simulink model "NE_Red_Rooster_Delta_B_28may"  (R2019b)
settings: Solver=FixedStepAuto  StartTime=0.0  StopTime=inf  FixedStep=0.0005  RelTol=1e-3
PreLoadFcn:
  | waijung.modelPreload; % Required for working with Waijung Blockset. Do not remove.
undefined symbols (not defined in the file): ARM, DiscIntNeverNeededParam, HSEOSC, Link, LQFP100, MDK, ST, STM32F407VG
libraries: simulink x30, stm32f4_i2c_lib x22, stm32f4_io_lib x6, stm32f4_reset_lib x1, stm32f4_device_config_lib x1
(part 3 of 5)

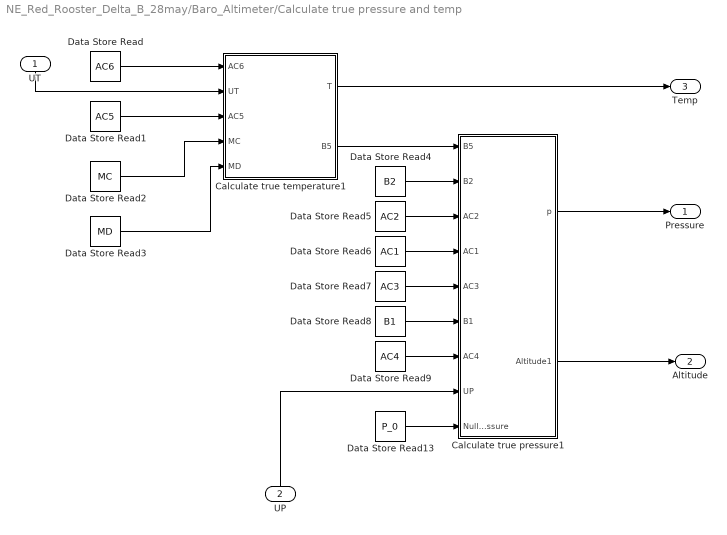
== system NE_Red_Rooster_Delta_B_28may/Baro_Altimeter/Calculate true pressure and temp  ==
  UT : Inport
  "UP " : Inport  Port=2
  Calculate true pressure1 : Subsystem
  Calculate true temperature1 : Subsystem
  Data Store Read : DataStoreRead  DataStoreName=AC6
  Data Store Read1 : DataStoreRead  DataStoreName=AC5
  Data Store Read13 : DataStoreRead  DataStoreName=P_0
  Data Store Read2 : DataStoreRead  DataStoreName=MC
  Data Store Read3 : DataStoreRead  DataStoreName=MD
  Data Store Read4 : DataStoreRead  DataStoreName=B2
  Data Store Read5 : DataStoreRead  DataStoreName=AC2
  Data Store Read6 : DataStoreRead  DataStoreName=AC1
  Data Store Read7 : DataStoreRead  DataStoreName=AC3
  Data Store Read8 : DataStoreRead  DataStoreName=B1
  Data Store Read9 : DataStoreRead  DataStoreName=AC4
  Pressure : Outport
  Altitude : Outport  Port=2
  "Temp " : Outport  Port=3
  wires:
  Calculate true temperature1/2(B5) -> Calculate true pressure1/1(B5)
  Calculate true pressure1/1(p) -> Pressure/1
  Calculate true pressure1/2(Altitude1) -> Altitude/1
  Data Store Read/1 -> Calculate true temperature1/1(AC6)
  Data Store Read1/1 -> Calculate true temperature1/3(AC5)
  Data Store Read2/1 -> Calculate true temperature1/4(MC)
  Data Store Read3/1 -> Calculate true temperature1/5(MD)
  Data Store Read4/1 -> Calculate true pressure1/2(B2)
  Data Store Read5/1 -> Calculate true pressure1/3(AC2)
  Data Store Read6/1 -> Calculate true pressure1/4(AC1)
  Data Store Read7/1 -> Calculate true pressure1/5(AC3)
  Data Store Read8/1 -> Calculate true pressure1/6(B1)
  Data Store Read9/1 -> Calculate true pressure1/7(AC4)
  Calculate true temperature1/1(T) -> "Temp "/1
  Data Store Read13/1 -> Calculate true pressure1/9("Null_Pressure ")
  "UP "/1 -> Calculate true pressure1/8(UP)
  UT/1 -> Calculate true temperature1/2(UT)

== system NE_Red_Rooster_Delta_B_28may/Baro_Altimeter/Read Pressure and Temp ==
  Constant : Constant  Value=hex2dec('EE')  OutDataTypeStr=uint8  SampleTime=-1
  Constant1 : Constant  Value=hex2dec('F4')  OutDataTypeStr=uint8  SampleTime=-1
  Constant4 : Constant  Value=hex2dec('2E')  OutDataTypeStr=uint8  SampleTime=-1
  Constant7 : Constant  Value=hex2dec('B4')  OutDataTypeStr=uint8  SampleTime=-1
  I2C Master Read/Write : stm32f4_i2c_lib/I2C Master Read//Write  configuration=Transaction  module=1  lastmodule=3  transfer=Blocking  dutycycle=TLow/THigh = 2  clkspeed=400  timeout=25  writecount=2  readcount=0  sdapin=C9  sclpin=A8  waitwritetime=14  forcestop=off  inputtypearray=[3 3 3 3]  outputtypearray=[1 3]  confstr="[\"C\",\"9\",\"A\",\"8\",\"1\",\"1\",\"6\",\"0\",\"I2C_DutyCycle_2\",\"14\",\"off\"]"  sampletime=-1  sampletimestr=-1  blockid=Baro_AltimeterReadPressureandTempI2CMasterReadWrite
  I2C Master Read/Write1 : stm32f4_i2c_lib/I2C Master Read//Write  configuration=Transaction  module=1  lastmodule=3  transfer=Blocking  dutycycle=TLow/THigh = 2  clkspeed=400  timeout=25  writecount=2  readcount=0  sdapin=C9  sclpin=A8  waitwritetime=5  forcestop=off  inputtypearray=[3 3 3 3]  outputtypearray=[1 3]  confstr="[\"C\",\"9\",\"A\",\"8\",\"1\",\"1\",\"6\",\"0\",\"I2C_DutyCycle_2\",\"5\",\"off\"]"  sampletime=-1  sampletimestr=-1  blockid=Baro_AltimeterReadPressureandTempI2CMasterReadWrite1
  If : If  IfExpression=u1 == 0  ShowElse=off
  If Action Subsystem : Subsystem  TreatAsAtomicUnit=on
  If Action Subsystem2 : Subsystem  TreatAsAtomicUnit=on
  If2 : If  IfExpression=u1 == 0  ShowElse=off
  UT : Outport
  UP : Outport  Port=2  OutDataTypeStr=uint32
  wires:
  Constant4/1 -> I2C Master Read/Write1/3
  If/1 -> If Action Subsystem/Action
  I2C Master Read/Write1/1 -> If/1
  If2/1 -> If Action Subsystem2/Action
  I2C Master Read/Write/1 -> If2/1
  Constant/1 -> I2C Master Read/Write/1, I2C Master Read/Write1/1
  Constant1/1 -> I2C Master Read/Write/2, I2C Master Read/Write1/2
  Constant7/1 -> I2C Master Read/Write/3
  If Action Subsystem2/1(Out1) -> UP/1
  If Action Subsystem/1(Out1) -> UT/1

== system NE_Red_Rooster_Delta_B_28may/Baro_Altimeter/Subsystem1 ==
  In1 : Inport
  Enable : EnablePort
  Constant : Constant  Value=0
  Data Store Write : DataStoreWrite  DataStoreName=P_0
  Data Store Write1 : DataStoreWrite
  wires:
  Constant/1 -> Data Store Write1/1
  In1/1 -> Data Store Write/1

== system NE_Red_Rooster_Delta_B_28may/Calibration data/Read calibration data  ==
  Subsystem_get_AC : Subsystem
  Subsystem_get_B : Subsystem
  Subsystem_get_M : Subsystem
  AC1 : Outport  OutDataTypeStr=int32
  AC2 : Outport  Port=2  OutDataTypeStr=int32
  AC3 : Outport  Port=3  OutDataTypeStr=int32
  AC4 : Outport  Port=4  OutDataTypeStr=uint32
  AC5 : Outport  Port=5  OutDataTypeStr=uint32
  AC6 : Outport  Port=6
  B1 : Outport  Port=7  OutDataTypeStr=int32
  B2 : Outport  Port=8  OutDataTypeStr=int32
  MB : Outport  Port=9  OutDataTypeStr=int32
  MC : Outport  Port=10  OutDataTypeStr=int32
  MD : Outport  Port=11  OutDataTypeStr=int32
  wires:
  Subsystem_get_M/1(MB) -> MB/1
  Subsystem_get_M/2(MC) -> MC/1
  Subsystem_get_M/3(MD) -> MD/1
  Subsystem_get_B/1(B1) -> B1/1
  Subsystem_get_B/2(B2) -> B2/1
  Subsystem_get_AC/6(AC6) -> AC6/1
  Subsystem_get_AC/5(AC5) -> AC5/1
  Subsystem_get_AC/4(AC4) -> AC4/1
  Subsystem_get_AC/3(AC3) -> AC3/1
  Subsystem_get_AC/2(AC2) -> AC2/1
  Subsystem_get_AC/1(AC1) -> AC1/1

== system NE_Red_Rooster_Delta_B_28may/Elevons_Throttle_PWM/If Action Subsystem ==
  In1 : Inport
  In2 : Inport  Port=2
  In3 : Inport  Port=3
  Action Port : ActionPort  ActionPortLabel=if { }
  Out1 : Outport
  Out2 : Outport  Port=2
  Out3 : Outport  Port=3
  wires:
  In1/1 -> Out1/1
  In2/1 -> Out2/1
  In3/1 -> Out3/1

== system NE_Red_Rooster_Delta_B_28may/Elevons_Throttle_PWM/If Action Subsystem2 ==
  In1 : Inport
  In2 : Inport  Port=2
  In3 : Inport  Port=3
  Action Port : ActionPort  ActionPortLabel=if { }
  Out1 : Outport
  Out2 : Outport  Port=2
  Out3 : Outport  Port=3
  wires:
  In1/1 -> Out1/1
  In2/1 -> Out2/1
  In3/1 -> Out3/1

== system NE_Red_Rooster_Delta_B_28may/Elevons_Throttle_PWM/If Action Subsystem3 ==
  In1 : Inport
  In2 : Inport  Port=2
  In3 : Inport  Port=3
  Action Port : ActionPort  ActionPortLabel=if { }
  Out1 : Outport
  Out2 : Outport  Port=2
  Out3 : Outport  Port=3
  wires:
  In3/1 -> Out3/1
  In2/1 -> Out2/1
  In1/1 -> Out1/1

== system NE_Red_Rooster_Delta_B_28may/Init_ADXL345/Subsystem ==
  Enable : EnablePort
  Constant : Constant
  Out1 : Outport
  wires:
  Constant/1 -> Out1/1

== system NE_Red_Rooster_Delta_B_28may/Init_L3GD4200 /Get Init L3G4200D1 ==
  SlvAddr : Inport
  Bitwise Operator : simulink/Logic and Bit Operations/Bitwise Operator  logicop=AND  UseBitMask=off  NumInputPorts=4  BitMask=bin2dec('11011001')  BitMaskRealWorld=Stored Integer
  CNTRL_REG1 : Constant  Value=hex2dec('20')  OutDataTypeStr=uint8  SampleTime=-1
  CNTRL_REG4 : Constant  Value=hex2dec('23')  OutDataTypeStr=uint8  SampleTime=-1
  Compare To Constant : simulink/Logic and Bit Operations/Compare To Constant  relop===  const=0  OutDataTypeStr=uint8  ZeroCross=off
  Compare To Constant1 : simulink/Logic and Bit Operations/Compare To Constant  relop===  const=hex2dec('0F')  OutDataTypeStr=uint8  ZeroCross=off
  Compare To Constant2 : simulink/Logic and Bit Operations/Compare To Constant  relop===  const=0  OutDataTypeStr=uint8  ZeroCross=off
  Compare To Constant3 : simulink/Logic and Bit Operations/Compare To Constant  relop===  const=0  OutDataTypeStr=uint8  ZeroCross=off
  I2C Master Read/Write : S-Function  FunctionName=stm32f4_i2c  Parameters=configuration,module,transfer,clkspeed,timeout,sdapin,sclpin,writecount,readcount,inputtypearray,outputtypearray,confstr,sampletime,sampletimestr,blockid  SFunctionDeploymentMode=off  EnableBusSupport=off  mask(stm32f4_i2c){configuration=Transaction, module=1, lastmodule=3, transfer=Blocking, dutycycle=TLow/THigh = 2, clkspeed=400, timeout=25, writecount=1, readcount=1, sdapin=C9, sclpin=A8, waitwritetime=0, inputtypearray=[2 3 3], outputtypearray=[2 3 3], confstr=["C","9","A","8","1","1","6","0","I2C_DutyCycle_2","0","off"], sampletime=-1, sampletimestr=0.0005, blockid=Init_L3GD4200GetInitL3G4200D1I2CMasterReadWrite}
      mask prompts: module "I2C Module"; lastmodule "Last module"; transfer "Transfer mode"; dutycycle "Duty cycle in fast mode"; clkspeed "Clock speed (kHz)"; timeout "Timeout (ms)"; writecount "Bytes write count"; readcount "Bytes read count"; sdapin "SDA pin"; sclpin "SCL pin"; waitwritetime "Wait write time (ms), default is 0"; inputtypearray "Input type array"; outputtypearray "Output type array"; confstr "Configuration string"; sampletime "Sample time (sec)"; sampletimestr "Compiled sample time (sec) in string"
      mask init:
      | stm32f4_i2c_callback('init');
      mask Help: web(fullfile(waijungdocroot,'stm32f4_i2c.htm'), '-browser')
      mask TypeOptions configuration: Setup | Transaction
      mask Callback configuration: stm32f4_i2c_callback('configuration');
      mask TypeOptions module: 1 | 2 | 3
      mask Callback module: stm32f4_i2c_callback('module');
      mask TypeOptions transfer: Blocking | Non-blocking
      mask TypeOptions dutycycle: TLow/THigh = 16/9 | TLow/THigh = 2
      mask Callback dutycycle: stm32f4_i2c_callback('dutycycle');
      mask Callback writecount: stm32f4_i2c_callback('writecount');
      mask Callback readcount: stm32f4_i2c_callback('readcount');
      mask TypeOptions sdapin: - | C9
      mask Callback sdapin: stm32f4_i2c_callback('sdapin');
      mask TypeOptions sclpin: - | A8
      mask Callback sclpin: stm32f4_i2c_callback('sclpin');
      mask Callback confstr: stm32f4_i2c_callback('confstr');
      mask Callback sampletime: stm32f4_i2c_callback('sampletime');
      mask Callback sampletimestr: stm32f4_i2c_callback('sampletimestr');
      mask Callback blockid: stm32f4_i2c_callback('blockid');
      mask Display: text(0.5, 0.5, 'Module: I2C1\nTransfer: Blocking\nWrite: 1 bytes\nRead: 1 bytes\nTs (sec): 0.0005','ver','middle','hor','center');port_label('input', 1,'SlvAddr');port_label('input', 2,'Wr0 (uint8)');port_label('output', 1,'Status');port_label('output', 2,'Rd0 (uint8)');
  I2C Master Read/Write1 : S-Function  FunctionName=stm32f4_i2c  Parameters=configuration,module,transfer,clkspeed,timeout,sdapin,sclpin,writecount,readcount,inputtypearray,outputtypearray,confstr,sampletime,sampletimestr,blockid  SFunctionDeploymentMode=off  EnableBusSupport=off  mask(stm32f4_i2c){configuration=Transaction, module=1, lastmodule=3, transfer=Blocking, dutycycle=TLow/THigh = 2, clkspeed=400, timeout=25, writecount=1, readcount=1, sdapin=C9, sclpin=A8, waitwritetime=0, inputtypearray=[2 3 3], outputtypearray=[2 3 3], confstr=["C","9","A","8","1","1","6","0","I2C_DutyCycle_2","0","off"], sampletime=-1, sampletimestr=0.0005, blockid=Init_L3GD4200GetInitL3G4200D1I2CMasterReadWrite1}
      mask prompts: module "I2C Module"; lastmodule "Last module"; transfer "Transfer mode"; dutycycle "Duty cycle in fast mode"; clkspeed "Clock speed (kHz)"; timeout "Timeout (ms)"; writecount "Bytes write count"; readcount "Bytes read count"; sdapin "SDA pin"; sclpin "SCL pin"; waitwritetime "Wait write time (ms), default is 0"; inputtypearray "Input type array"; outputtypearray "Output type array"; confstr "Configuration string"; sampletime "Sample time (sec)"; sampletimestr "Compiled sample time (sec) in string"
      mask init:
      | stm32f4_i2c_callback('init');
      mask Help: web(fullfile(waijungdocroot,'stm32f4_i2c.htm'), '-browser')
      mask TypeOptions configuration: Setup | Transaction
      mask Callback configuration: stm32f4_i2c_callback('configuration');
      mask TypeOptions module: 1 | 2 | 3
      mask Callback module: stm32f4_i2c_callback('module');
      mask TypeOptions transfer: Blocking | Non-blocking
      mask TypeOptions dutycycle: TLow/THigh = 16/9 | TLow/THigh = 2
      mask Callback dutycycle: stm32f4_i2c_callback('dutycycle');
      mask Callback writecount: stm32f4_i2c_callback('writecount');
      mask Callback readcount: stm32f4_i2c_callback('readcount');
      mask TypeOptions sdapin: - | C9
      mask Callback sdapin: stm32f4_i2c_callback('sdapin');
      mask TypeOptions sclpin: - | A8
      mask Callback sclpin: stm32f4_i2c_callback('sclpin');
      mask Callback confstr: stm32f4_i2c_callback('confstr');
      mask Callback sampletime: stm32f4_i2c_callback('sampletime');
      mask Callback sampletimestr: stm32f4_i2c_callback('sampletimestr');
      mask Callback blockid: stm32f4_i2c_callback('blockid');
      mask Display: text(0.5, 0.5, 'Module: I2C1\nTransfer: Blocking\nWrite: 1 bytes\nRead: 1 bytes\nTs (sec): 0.0005','ver','middle','hor','center');port_label('input', 1,'SlvAddr');port_label('input', 2,'Wr0 (uint8)');port_label('output', 1,'Status');port_label('output', 2,'Rd0 (uint8)');
  Initial Done : Outport
  wires:
  Compare To Constant3/1 -> Bitwise Operator/4
  Compare To Constant2/1 -> Bitwise Operator/3
  Compare To Constant1/1 -> Bitwise Operator/2
  Compare To Constant/1 -> Bitwise Operator/1
  Bitwise Operator/1 -> Initial Done/1
  I2C Master Read/Write1/2 -> Compare To Constant3/1
  I2C Master Read/Write1/1 -> Compare To Constant2/1
  I2C Master Read/Write/2 -> Compare To Constant1/1
  I2C Master Read/Write/1 -> Compare To Constant/1
  SlvAddr/1 -> I2C Master Read/Write/1, I2C Master Read/Write1/1
  CNTRL_REG1/1 -> I2C Master Read/Write/2
  CNTRL_REG4/1 -> I2C Master Read/Write1/2

== system NE_Red_Rooster_Delta_B_28may/Init_L3GD4200 /Init L3G4200D ==
  Enable1 : EnablePort  PropagateVarSize=During execution
  Bitwise Operator : simulink/Logic and Bit Operations/Bitwise Operator  logicop=AND  UseBitMask=off  NumInputPorts=2  BitMask=bin2dec('11011001')  BitMaskRealWorld=Stored Integer
  CNTRL_REG1 : Constant  Value=hex2dec('20')  OutDataTypeStr=uint8  SampleTime=-1
  CNTRL_REG4 : Constant  Value=hex2dec('23')  OutDataTypeStr=uint8  SampleTime=-1
  Compare To Zero : simulink/Logic and Bit Operations/Compare To Zero  relop===  OutDataTypeStr=boolean
  Compare To Zero1 : simulink/Logic and Bit Operations/Compare To Zero  relop===  OutDataTypeStr=boolean
  Enable : Constant  Value=hex2dec('0F')  OutDataTypeStr=uint8  SampleTime=-1
  FS 250 : Constant  Value=hex2dec('00')  OutDataTypeStr=uint8  SampleTime=-1
  I2C Master Read/Write : S-Function  FunctionName=stm32f4_i2c  Parameters=configuration,module,transfer,clkspeed,timeout,sdapin,sclpin,writecount,readcount,inputtypearray,outputtypearray,confstr,sampletime,sampletimestr,blockid  SFunctionDeploymentMode=off  EnableBusSupport=off  mask(stm32f4_i2c){configuration=Transaction, module=1, lastmodule=3, transfer=Blocking, dutycycle=TLow/THigh = 2, clkspeed=400, timeout=25, writecount=2, readcount=0, sdapin=C9, sclpin=A8, waitwritetime=0, inputtypearray=[3 3 3 3], outputtypearray=[1 3], confstr=["C","9","A","8","1","1","6","0","I2C_DutyCycle_2","0","off"], sampletime=-1, sampletimestr=0.0005, blockid=Init_L3GD4200InitL3G4200DI2CMasterReadWrite}
      mask prompts: module "I2C Module"; lastmodule "Last module"; transfer "Transfer mode"; dutycycle "Duty cycle in fast mode"; clkspeed "Clock speed (kHz)"; timeout "Timeout (ms)"; writecount "Bytes write count"; readcount "Bytes read count"; sdapin "SDA pin"; sclpin "SCL pin"; waitwritetime "Wait write time (ms), default is 0"; inputtypearray "Input type array"; outputtypearray "Output type array"; confstr "Configuration string"; sampletime "Sample time (sec)"; sampletimestr "Compiled sample time (sec) in string"
      mask init:
      | stm32f4_i2c_callback('init');
      mask Help: web(fullfile(waijungdocroot,'stm32f4_i2c.htm'), '-browser')
      mask TypeOptions configuration: Setup | Transaction
      mask Callback configuration: stm32f4_i2c_callback('configuration');
      mask TypeOptions module: 1 | 2 | 3
      mask Callback module: stm32f4_i2c_callback('module');
      mask TypeOptions transfer: Blocking | Non-blocking
      mask TypeOptions dutycycle: TLow/THigh = 16/9 | TLow/THigh = 2
      mask Callback dutycycle: stm32f4_i2c_callback('dutycycle');
      mask Callback writecount: stm32f4_i2c_callback('writecount');
      mask Callback readcount: stm32f4_i2c_callback('readcount');
      mask TypeOptions sdapin: - | C9
      mask Callback sdapin: stm32f4_i2c_callback('sdapin');
      mask TypeOptions sclpin: - | A8
      mask Callback sclpin: stm32f4_i2c_callback('sclpin');
      mask Callback confstr: stm32f4_i2c_callback('confstr');
      mask Callback sampletime: stm32f4_i2c_callback('sampletime');
      mask Callback sampletimestr: stm32f4_i2c_callback('sampletimestr');
      mask Callback blockid: stm32f4_i2c_callback('blockid');
      mask Display: text(0.5, 0.5, 'Module: I2C1\nTransfer: Blocking\nWrite: 2 bytes\nRead: 0 bytes\nTs (sec): 0.0005','ver','middle','hor','center');port_label('input', 1,'SlvAddr');port_label('input', 2,'Wr0 (uint8)');port_label('input', 3,'Wr1 (uint8)');port_label('output', 1,'Status');
  I2C Master Read/Write1 : S-Function  FunctionName=stm32f4_i2c  Parameters=configuration,module,transfer,clkspeed,timeout,sdapin,sclpin,writecount,readcount,inputtypearray,outputtypearray,confstr,sampletime,sampletimestr,blockid  SFunctionDeploymentMode=off  EnableBusSupport=off  mask(stm32f4_i2c){configuration=Transaction, module=1, lastmodule=3, transfer=Blocking, dutycycle=TLow/THigh = 2, clkspeed=400, timeout=25, writecount=2, readcount=0, sdapin=C9, sclpin=A8, waitwritetime=0, inputtypearray=[3 3 3 3], outputtypearray=[1 3], confstr=["C","9","A","8","1","1","6","0","I2C_DutyCycle_2","0","off"], sampletime=-1, sampletimestr=0.0005, blockid=Init_L3GD4200InitL3G4200DI2CMasterReadWrite1}
      mask prompts: module "I2C Module"; lastmodule "Last module"; transfer "Transfer mode"; dutycycle "Duty cycle in fast mode"; clkspeed "Clock speed (kHz)"; timeout "Timeout (ms)"; writecount "Bytes write count"; readcount "Bytes read count"; sdapin "SDA pin"; sclpin "SCL pin"; waitwritetime "Wait write time (ms), default is 0"; inputtypearray "Input type array"; outputtypearray "Output type array"; confstr "Configuration string"; sampletime "Sample time (sec)"; sampletimestr "Compiled sample time (sec) in string"
      mask init:
      | stm32f4_i2c_callback('init');
      mask Help: web(fullfile(waijungdocroot,'stm32f4_i2c.htm'), '-browser')
      mask TypeOptions configuration: Setup | Transaction
      mask Callback configuration: stm32f4_i2c_callback('configuration');
      mask TypeOptions module: 1 | 2 | 3
      mask Callback module: stm32f4_i2c_callback('module');
      mask TypeOptions transfer: Blocking | Non-blocking
      mask TypeOptions dutycycle: TLow/THigh = 16/9 | TLow/THigh = 2
      mask Callback dutycycle: stm32f4_i2c_callback('dutycycle');
      mask Callback writecount: stm32f4_i2c_callback('writecount');
      mask Callback readcount: stm32f4_i2c_callback('readcount');
      mask TypeOptions sdapin: - | C9
      mask Callback sdapin: stm32f4_i2c_callback('sdapin');
      mask TypeOptions sclpin: - | A8
      mask Callback sclpin: stm32f4_i2c_callback('sclpin');
      mask Callback confstr: stm32f4_i2c_callback('confstr');
      mask Callback sampletime: stm32f4_i2c_callback('sampletime');
      mask Callback sampletimestr: stm32f4_i2c_callback('sampletimestr');
      mask Callback blockid: stm32f4_i2c_callback('blockid');
      mask Display: text(0.5, 0.5, 'Module: I2C1\nTransfer: Blocking\nWrite: 2 bytes\nRead: 0 bytes\nTs (sec): 0.0005','ver','middle','hor','center');port_label('input', 1,'SlvAddr');port_label('input', 2,'Wr0 (uint8)');port_label('input', 3,'Wr1 (uint8)');port_label('output', 1,'Status');
  SlvAddr1 : Constant  Value=hex2dec('D2')  OutDataTypeStr=uint8  SampleTime=-1
  Subsystem : Subsystem
  Subsystem1 : Subsystem
  Terminator : Terminator
  wires:
  I2C Master Read/Write1/1 -> Compare To Zero1/1
  I2C Master Read/Write/1 -> Compare To Zero/1
  CNTRL_REG4/1 -> I2C Master Read/Write1/2
  FS 250/1 -> I2C Master Read/Write1/3
  Enable/1 -> I2C Master Read/Write/3
  CNTRL_REG1/1 -> I2C Master Read/Write/2
  SlvAddr1/1 -> I2C Master Read/Write1/1, I2C Master Read/Write/1
  Compare To Zero/1 -> Subsystem/Enable
  Compare To Zero1/1 -> Subsystem1/Enable
  Subsystem/1(Out1) -> Bitwise Operator/1
  Subsystem1/1(Out1) -> Bitwise Operator/2
  Bitwise Operator/1 -> Terminator/1

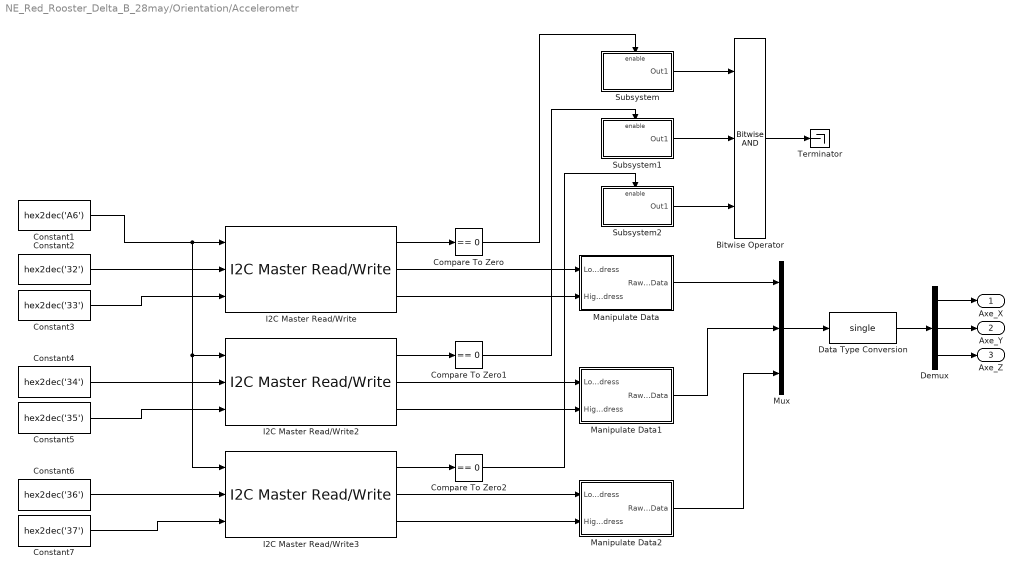
== system NE_Red_Rooster_Delta_B_28may/Orientation/Accelerometr ==
  Bitwise Operator : simulink/Logic and Bit Operations/Bitwise Operator  logicop=AND  UseBitMask=off  NumInputPorts=3  BitMask=bin2dec('11011001')  BitMaskRealWorld=Stored Integer
  Compare To Zero : simulink/Logic and Bit Operations/Compare To Zero  relop===  OutDataTypeStr=boolean
  Compare To Zero1 : simulink/Logic and Bit Operations/Compare To Zero  relop===  OutDataTypeStr=boolean
  Compare To Zero2 : simulink/Logic and Bit Operations/Compare To Zero  relop===  OutDataTypeStr=boolean
  Constant1 : Constant  Value=hex2dec('A6')  OutDataTypeStr=uint8  SampleTime=-1
  Constant2 : Constant  Value=hex2dec('32')  OutDataTypeStr=uint8  SampleTime=-1
  Constant3 : Constant  Value=hex2dec('33')  OutDataTypeStr=uint8  SampleTime=-1
  Constant4 : Constant  Value=hex2dec('34')  OutDataTypeStr=uint8  SampleTime=-1
  Constant5 : Constant  Value=hex2dec('35')  OutDataTypeStr=uint8  SampleTime=-1
  Constant6 : Constant  Value=hex2dec('36')  OutDataTypeStr=uint8  SampleTime=-1
  Constant7 : Constant  Value=hex2dec('37')  OutDataTypeStr=uint8  SampleTime=-1
  Data Type Conversion : DataTypeConversion  OutDataTypeStr=single
  Demux : Demux  Outputs=3
  I2C Master Read/Write : stm32f4_i2c_lib/I2C Master Read//Write  configuration=Transaction  module=1  lastmodule=3  transfer=Blocking  dutycycle=TLow/THigh = 2  clkspeed=400  timeout=25  writecount=2  readcount=2  sdapin=C9  sclpin=A8  waitwritetime=0  forcestop=off  inputtypearray=[3 3 3 3]  outputtypearray=[3 3 3 3]  confstr="[\"C\",\"9\",\"A\",\"8\",\"1\",\"1\",\"6\",\"0\",\"I2C_DutyCycle_2\",\"0\",\"off\"]"  sampletime=-1  sampletimestr=-1  blockid=OrientationAccelerometrI2CMasterReadWrite
  I2C Master Read/Write2 : stm32f4_i2c_lib/I2C Master Read//Write  configuration=Transaction  module=1  lastmodule=3  transfer=Blocking  dutycycle=TLow/THigh = 2  clkspeed=400  timeout=25  writecount=2  readcount=2  sdapin=C9  sclpin=A8  waitwritetime=0  forcestop=off  inputtypearray=[3 3 3 3]  outputtypearray=[3 3 3 3]  confstr="[\"C\",\"9\",\"A\",\"8\",\"1\",\"1\",\"6\",\"0\",\"I2C_DutyCycle_2\",\"0\",\"off\"]"  sampletime=-1  sampletimestr=-1  blockid=OrientationAccelerometrI2CMasterReadWrite2
  I2C Master Read/Write3 : stm32f4_i2c_lib/I2C Master Read//Write  configuration=Transaction  module=1  lastmodule=3  transfer=Blocking  dutycycle=TLow/THigh = 2  clkspeed=400  timeout=25  writecount=2  readcount=2  sdapin=C9  sclpin=A8  waitwritetime=0  forcestop=off  inputtypearray=[3 3 3 3]  outputtypearray=[3 3 3 3]  confstr="[\"C\",\"9\",\"A\",\"8\",\"1\",\"1\",\"6\",\"0\",\"I2C_DutyCycle_2\",\"0\",\"off\"]"  sampletime=-1  sampletimestr=-1  blockid=OrientationAccelerometrI2CMasterReadWrite3
  Manipulate Data : Subsystem
  Manipulate Data1 : Subsystem
  Manipulate Data2 : Subsystem
  Mux : Mux  Inputs=3
  Subsystem : Subsystem
  Subsystem1 : Subsystem
  Subsystem2 : Subsystem
  Terminator : Terminator
  Axe_X : Outport
  Axe_Y : Outport  Port=2
  Axe_Z : Outport  Port=3
  wires:
  I2C Master Read/Write3/2 -> Manipulate Data2/1(LowAddress)
  I2C Master Read/Write2/3 -> Manipulate Data1/2(HighAddress)
  I2C Master Read/Write/1 -> Compare To Zero/1
  Constant7/1 -> I2C Master Read/Write3/3
  I2C Master Read/Write3/3 -> Manipulate Data2/2(HighAddress)
  Mux/1 -> Data Type Conversion/1
  Constant4/1 -> I2C Master Read/Write2/2
  Constant1/1 -> I2C Master Read/Write3/1, I2C Master Read/Write2/1, I2C Master Read/Write/1
  I2C Master Read/Write2/2 -> Manipulate Data1/1(LowAddress)
  I2C Master Read/Write/3 -> Manipulate Data/2(HighAddress)
  I2C Master Read/Write3/1 -> Compare To Zero2/1
  Constant6/1 -> I2C Master Read/Write3/2
  Manipulate Data2/1(RawAccData) -> Mux/3
  Constant5/1 -> I2C Master Read/Write2/3
  Manipulate Data1/1(RawAccData) -> Mux/2
  I2C Master Read/Write/2 -> Manipulate Data/1(LowAddress)
  Constant2/1 -> I2C Master Read/Write/2
  Constant3/1 -> I2C Master Read/Write/3
  I2C Master Read/Write2/1 -> Compare To Zero1/1
  Manipulate Data/1(RawAccData) -> Mux/1
  Compare To Zero/1 -> Subsystem/Enable
  Compare To Zero1/1 -> Subsystem1/Enable
  Compare To Zero2/1 -> Subsystem2/Enable
  Data Type Conversion/1 -> Demux/1
  Demux/2 -> Axe_Y/1
  Demux/1 -> Axe_X/1
  Demux/3 -> Axe_Z/1
  Subsystem/1(Out1) -> Bitwise Operator/1
  Subsystem1/1(Out1) -> Bitwise Operator/2
  Subsystem2/1(Out1) -> Bitwise Operator/3
  Bitwise Operator/1 -> Terminator/1

== system NE_Red_Rooster_Delta_B_28may/Orientation/Gyro ==
  Compare To Zero1 : simulink/Logic and Bit Operations/Compare To Zero  relop===  OutDataTypeStr=boolean  ZeroCross=off
  Data_transformation : Subsystem
  L3G4200D : Subsystem
  Success : Subsystem
      mask Display: image('C:\Users\Alexander Gorbunov\Pictures\Roll_Pitch_Yaw.JPG');
  Out1 : Outport
  Out2 : Outport  Port=2
  Out3 : Outport  Port=3
  wires:
  Success/1(Gyr_X) -> Data_transformation/1(In1)
  L3G4200D/1(Status) -> Compare To Zero1/1
  L3G4200D/4(Z) -> Success/3(In3)
  L3G4200D/3(Y) -> Success/2(In2)
  Success/2(Gyr_Y) -> Data_transformation/2(In2)
  Success/3(Gyr_Z) -> Data_transformation/3(In3)
  L3G4200D/2(X) -> Success/1(In1)
  Compare To Zero1/1 -> Success/Enable
  Data_transformation/1(Out1) -> Out1/1
  Data_transformation/2(Out2) -> Out2/1
  Data_transformation/3(Out3) -> Out3/1

== system NE_Red_Rooster_Delta_B_28may/Orientation/KREN ==
  Za_F : Inport
  Xa_F : Inport  Port=2
  Ya_F : Inport  Port=3
  Add : Sum
  Constant : Constant  Value=57.23
  Divide : Product  Inputs=*/
  Math Function : Math  Operator=square  SaturateOnIntegerOverflow=on
  Math Function1 : Math  Operator=square  SaturateOnIntegerOverflow=on
  Product : Product
  Sqrt : Sqrt  SaturateOnIntegerOverflow=on
  Trigonometric Function : Trigonometry  Operator=atan
  ACC_Roll : Outport
  wires:
  Sqrt/1 -> Divide/2
  Za_F/1 -> Math Function/1
  Ya_F/1 -> Divide/1
  Xa_F/1 -> Math Function1/1
  Add/1 -> Sqrt/1
  Trigonometric Function/1 -> Product/1
  Divide/1 -> Trigonometric Function/1
  Math Function/1 -> Add/1
  Math Function1/1 -> Add/2
  Constant/1 -> Product/2
  Product/1 -> ACC_Roll/1

== system NE_Red_Rooster_Delta_B_28may/Orientation/KREN_RESULT_ANG ==
  Gyr_Data : Inport
  Acc_Data : Inport  Port=2
  Add : Sum
  Add1 : Sum
  Constant : Constant  Value=0.02
  Constant1 : Constant  Value=4.1
  Constant2 : Constant  Value=0.05
  Divide : Product  Inputs=*/
  Product : Product
  Product1 : Product
  Sum : Sum  Inputs=|++
  Out1 : Outport
  wires:
  Acc_Data/1 -> Product1/2
  Constant/1 -> Add/1, Product/2
  Product/1 -> Sum/1
  Product1/1 -> Sum/2
  Constant2/1 -> Add/2, Product1/1
  Gyr_Data/1 -> Product/1
  Sum/1 -> Divide/1
  Add/1 -> Divide/2
  Divide/1 -> Add1/1
  Add1/1 -> Out1/1

== system NE_Red_Rooster_Delta_B_28may/Orientation/TANGASCH ==
  Za_F : Inport
  Ya_F : Inport  Port=2
  Xa_F : Inport  Port=3
  Add : Sum
  Constant : Constant  Value=57.23
  Divide : Product  Inputs=*/
  Math Function : Math  Operator=square  SaturateOnIntegerOverflow=on
  Math Function1 : Math  Operator=square  SaturateOnIntegerOverflow=on
  Product : Product
  Sqrt : Sqrt  SaturateOnIntegerOverflow=on
  Trigonometric Function : Trigonometry  Operator=atan
  ACC_Pitch : Outport
  wires:
  Math Function1/1 -> Add/2
  Math Function/1 -> Add/1
  Divide/1 -> Trigonometric Function/1
  Trigonometric Function/1 -> Product/1
  Add/1 -> Sqrt/1
  Ya_F/1 -> Math Function1/1
  Xa_F/1 -> Divide/1
  Za_F/1 -> Math Function/1
  Sqrt/1 -> Divide/2
  Constant/1 -> Product/2
  Product/1 -> ACC_Pitch/1

== system NE_Red_Rooster_Delta_B_28may/Orientation/TANGASCH_RESULT_ANG ==
  Gyr_Data : Inport
  Acc_Data : Inport  Port=2
  Add : Sum
  Add1 : Sum
  Constant : Constant  Value=0.02
  Constant1 : Constant  Value=0
  Constant2 : Constant  Value=0.05
  Divide : Product  Inputs=*/
  Product : Product
  Product1 : Product
  Sum : Sum  Inputs=|++
  Out1 : Outport
  wires:
  Constant1/1 -> Add1/2
  Add1/1 -> Out1/1
  Divide/1 -> Add1/1
  Add/1 -> Divide/2
  Sum/1 -> Divide/1
  Gyr_Data/1 -> Product/1
  Constant2/1 -> Product1/1, Add/2
  Product1/1 -> Sum/2
  Product/1 -> Sum/1
  Constant/1 -> Product/2, Add/1
  Acc_Data/1 -> Product1/2

== system NE_Red_Rooster_Delta_B_28may/Reset_Subsystem/Enabled Subsystem ==
  Enable : EnablePort
  System Reset : stm32f4_reset_lib/System Reset  conf=<empty>  sampletime=-1  sampletimestr=0.0005  blockid=Reset_SubsystemEnabledSubsystemSystemReset  inputarray=[]  inputlabelarray={}  outputarray=[]  outputlabelarray={}  compat=0  confstr="[\"Param1\",\"Param1\"]"

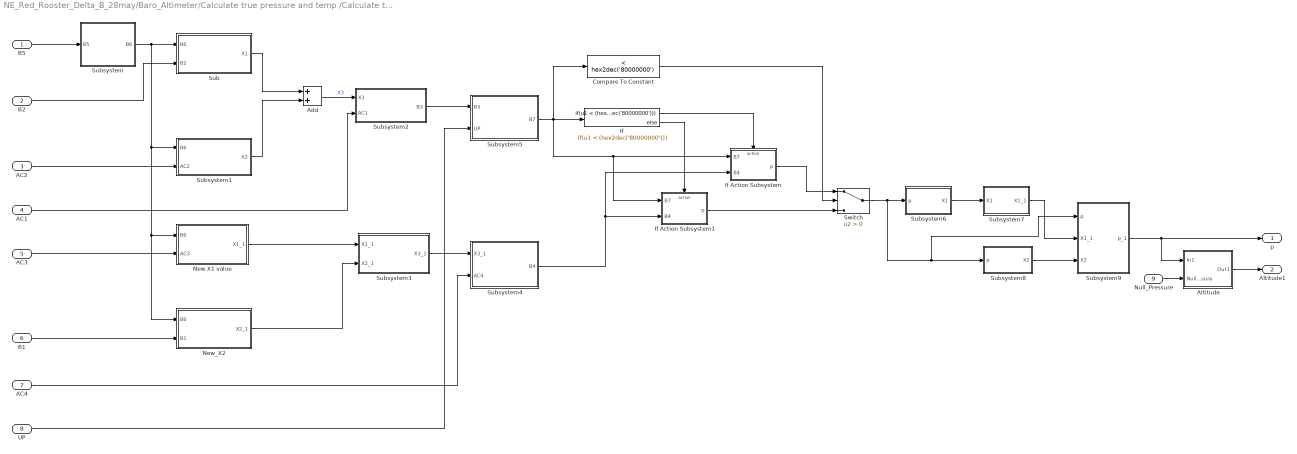
== system NE_Red_Rooster_Delta_B_28may/Baro_Altimeter/Calculate true pressure and temp /Calculate true pressure1 ==
  B5 : Inport
  B2 : Inport  Port=2
  AC2 : Inport  Port=3
  AC1 : Inport  Port=4
  AC3 : Inport  Port=5
  B1 : Inport  Port=6
  AC4 : Inport  Port=7
  UP : Inport  Port=8
  "Null_Pressure " : Inport  Port=9
  Add : Sum  OutDataTypeStr=int32
  Altitude : Subsystem
  Compare To Constant : simulink/Logic and Bit Operations/Compare To Constant  relop=<  const=hex2dec('80000000')  OutDataTypeStr=boolean
  If : If  IfExpression=u1 < (hex2dec('80000000'))
  If Action Subsystem : Subsystem  TreatAsAtomicUnit=on
  If Action Subsystem1 : Subsystem  TreatAsAtomicUnit=on
  New X1 value : Subsystem
  New_X2 : Subsystem
  Sub : Subsystem
  Subsystem : Subsystem
  Subsystem1 : Subsystem
  Subsystem2 : Subsystem
  Subsystem3 : Subsystem
  Subsystem4 : Subsystem
  Subsystem5 : Subsystem
  Subsystem6 : Subsystem
  Subsystem7 : Subsystem
  Subsystem8 : Subsystem
  Subsystem9 : Subsystem
  Switch : Switch  Criteria=u2 > Threshold
  p : Outport
  Altitude1 : Outport  Port=2  OutDataTypeStr=single
  wires:
  B5/1 -> Subsystem/1(B5)
  Subsystem/1(B6) -> New_X2/1(B6), New X1 value/1(B6), Subsystem1/1(B6), Sub/1(B6)
  B2/1 -> Sub/2(B2)
  AC2/1 -> Subsystem1/2(AC2)
  Sub/1(X1) -> Add/1
  Subsystem1/1(X2) -> Add/2
  Add/1 -> Subsystem2/1(X3)  "X3"
  AC1/1 -> Subsystem2/2(AC1)
  AC3/1 -> New X1 value/2(AC3)
  B1/1 -> New_X2/2(B1)
  New X1 value/1(X1_1) -> Subsystem3/1(X1_1)
  New_X2/1(X2_1) -> Subsystem3/2(X2_1)
  Subsystem3/1(X3_1) -> Subsystem4/1(X3_1)
  AC4/1 -> Subsystem4/2(AC4)
  Subsystem2/1(B3) -> Subsystem5/1(B3)
  UP/1 -> Subsystem5/2(UP)
  Subsystem5/1(B7) -> Compare To Constant/1, If Action Subsystem1/1(B7), If Action Subsystem/1(B7), If/1
  If/2 -> If Action Subsystem1/Action
  Subsystem4/1(B4) -> If Action Subsystem/2(B4), If Action Subsystem1/2(B4)
  If Action Subsystem1/1(p) -> Switch/3
  Subsystem6/1(X1) -> Subsystem7/1(X1)
  Subsystem7/1(X1_1) -> Subsystem9/2(X1_1)
  Subsystem8/1(X2) -> Subsystem9/3(X2)
  Subsystem9/1(p_1) -> Altitude/1(In1), p/1
  Switch/1 -> Subsystem6/1(p), Subsystem8/1(p), Subsystem9/1(p)
  If Action Subsystem/1(p) -> Switch/1
  If/1 -> If Action Subsystem/Action
  Compare To Constant/1 -> Switch/2
  Altitude/1(Out1) -> Altitude1/1
  "Null_Pressure "/1 -> Altitude/2("Null_Pressure ")

== system NE_Red_Rooster_Delta_B_28may/Baro_Altimeter/Calculate true pressure and temp /Calculate true temperature1 ==
  note: B5
  AC6 : Inport
  UT : Inport  Port=2
  AC5 : Inport  Port=3
  MC : Inport  Port=4
  MD : Inport  Port=5
  Add : Sum  OutDataTypeStr=int32
  Subsystem : Subsystem
  Subsystem1 : Subsystem
  Subsystem2 : Subsystem
  T : Outport
  B5 : Outport  Port=2  OutDataTypeStr=int32
  wires:
  UT/1 -> Subsystem/1(UT)
  AC6/1 -> Subsystem/2(AC6)
  AC5/1 -> Subsystem/3(AC5)
  Subsystem/1(X1) -> Subsystem1/1(X1), Add/1
  MC/1 -> Subsystem1/2(MC)
  MD/1 -> Subsystem1/3(MD)
  Subsystem1/1(X2) -> Add/2
  Add/1 -> B5/1, Subsystem2/1(B5)
  Subsystem2/1(T) -> T/1

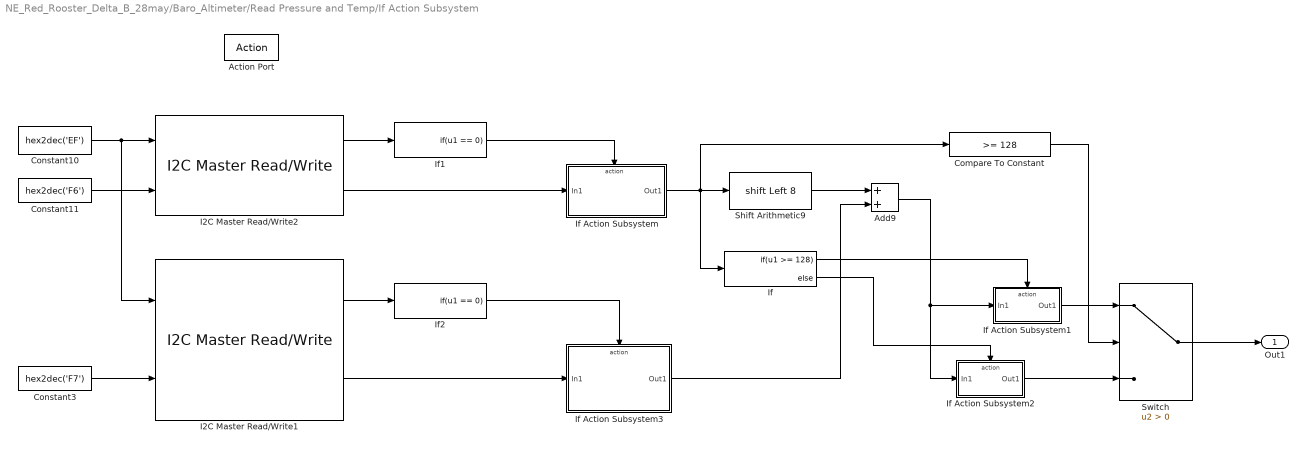
== system NE_Red_Rooster_Delta_B_28may/Baro_Altimeter/Read Pressure and Temp/If Action Subsystem ==
  Action Port : ActionPort  ActionPortLabel=if { }
  Add9 : Sum  AccumDataTypeStr=uint32  OutDataTypeStr=int32
  Compare To Constant : simulink/Logic and Bit Operations/Compare To Constant  relop=>=  const=128  OutDataTypeStr=boolean
  Constant10 : Constant  Value=hex2dec('EF')  OutDataTypeStr=uint8
  Constant11 : Constant  Value=hex2dec('F6')  OutDataTypeStr=uint8
  Constant3 : Constant  Value=hex2dec('F7')  OutDataTypeStr=uint8
  I2C Master Read/Write1 : stm32f4_i2c_lib/I2C Master Read//Write  configuration=Transaction  module=1  lastmodule=3  transfer=Blocking  dutycycle=TLow/THigh = 2  clkspeed=400  timeout=25  writecount=1  readcount=1  sdapin=C9  sclpin=A8  waitwritetime=0  forcestop=off  inputtypearray=[2 3 3]  outputtypearray=[2 3 3]  confstr="[\"C\",\"9\",\"A\",\"8\",\"1\",\"1\",\"6\",\"0\",\"I2C_DutyCycle_2\",\"0\",\"off\"]"  sampletime=-1  sampletimestr=Inf  blockid=Baro_AltimeterReadPressureandTempIfActionSubsystemI2CMasterReadWrite1
  I2C Master Read/Write2 : stm32f4_i2c_lib/I2C Master Read//Write  configuration=Transaction  module=1  lastmodule=3  transfer=Blocking  dutycycle=TLow/THigh = 2  clkspeed=400  timeout=25  writecount=1  readcount=1  sdapin=C9  sclpin=A8  waitwritetime=0  forcestop=off  inputtypearray=[2 3 3]  outputtypearray=[2 3 3]  confstr="[\"C\",\"9\",\"A\",\"8\",\"1\",\"1\",\"6\",\"0\",\"I2C_DutyCycle_2\",\"0\",\"off\"]"  sampletime=-1  sampletimestr=Inf  blockid=Baro_AltimeterReadPressureandTempIfActionSubsystemI2CMasterReadWrite2
  If : If  IfExpression=u1 >= 128
  If Action Subsystem : Subsystem  TreatAsAtomicUnit=on
  If Action Subsystem1 : Subsystem  TreatAsAtomicUnit=on
  If Action Subsystem2 : Subsystem  TreatAsAtomicUnit=on
  If Action Subsystem3 : Subsystem  TreatAsAtomicUnit=on
  If1 : If  IfExpression=u1 == 0  ShowElse=off
  If2 : If  IfExpression=u1 == 0  ShowElse=off
  Shift Arithmetic9 : ArithShift  BitShiftNumber=8  BitShiftDirection=Left
  Switch : Switch  Criteria=u2 > Threshold
  Out1 : Outport
  wires:
  Constant11/1 -> I2C Master Read/Write2/2
  I2C Master Read/Write2/1 -> If1/1
  If1/1 -> If Action Subsystem/Action
  Add9/1 -> If Action Subsystem2/1(In1), If Action Subsystem1/1(In1)
  Compare To Constant/1 -> Switch/2
  Shift Arithmetic9/1 -> Add9/1
  If Action Subsystem3/1(Out1) -> Add9/2
  If/1 -> If Action Subsystem1/Action
  If/2 -> If Action Subsystem2/Action
  If Action Subsystem1/1(Out1) -> Switch/1
  If Action Subsystem2/1(Out1) -> Switch/3
  Constant3/1 -> I2C Master Read/Write1/2
  I2C Master Read/Write1/1 -> If2/1
  If2/1 -> If Action Subsystem3/Action
  I2C Master Read/Write2/2 -> If Action Subsystem/1(In1)
  I2C Master Read/Write1/2 -> If Action Subsystem3/1(In1)
  Constant10/1 -> I2C Master Read/Write1/1, I2C Master Read/Write2/1
  If Action Subsystem/1(Out1) -> Compare To Constant/1, If/1, Shift Arithmetic9/1
  Switch/1 -> Out1/1

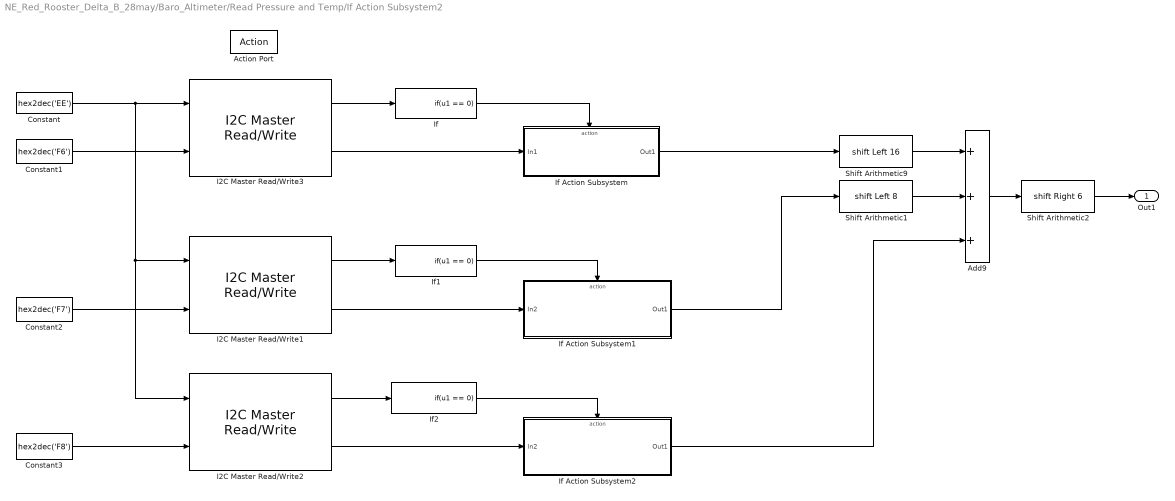
== system NE_Red_Rooster_Delta_B_28may/Baro_Altimeter/Read Pressure and Temp/If Action Subsystem2 ==
  Action Port : ActionPort  ActionPortLabel=if { }
  Add9 : Sum  Inputs=+++  AccumDataTypeStr=uint32  OutDataTypeStr=uint32
  Constant : Constant  Value=hex2dec('EE')  OutDataTypeStr=uint8
  Constant1 : Constant  Value=hex2dec('F6')  OutDataTypeStr=uint8
  Constant2 : Constant  Value=hex2dec('F7')  OutDataTypeStr=uint8
  Constant3 : Constant  Value=hex2dec('F8')  OutDataTypeStr=uint8
  I2C Master Read/Write1 : stm32f4_i2c_lib/I2C Master Read//Write  configuration=Transaction  module=1  lastmodule=3  transfer=Blocking  dutycycle=TLow/THigh = 2  clkspeed=400  timeout=25  writecount=1  readcount=1  sdapin=C9  sclpin=A8  waitwritetime=0  forcestop=on  inputtypearray=[2 3 3]  outputtypearray=[2 3 3]  confstr="[\"C\",\"9\",\"A\",\"8\",\"1\",\"1\",\"6\",\"0\",\"I2C_DutyCycle_2\",\"0\",\"on\"]"  sampletime=-1  sampletimestr=Inf  blockid=Baro_AltimeterReadPressureandTempIfActionSubsystem2I2CMasterReadWrite1
  I2C Master Read/Write2 : stm32f4_i2c_lib/I2C Master Read//Write  configuration=Transaction  module=1  lastmodule=3  transfer=Blocking  dutycycle=TLow/THigh = 2  clkspeed=400  timeout=25  writecount=1  readcount=1  sdapin=C9  sclpin=A8  waitwritetime=0  forcestop=on  inputtypearray=[2 3 3]  outputtypearray=[2 3 3]  confstr="[\"C\",\"9\",\"A\",\"8\",\"1\",\"1\",\"6\",\"0\",\"I2C_DutyCycle_2\",\"0\",\"on\"]"  sampletime=-1  sampletimestr=Inf  blockid=Baro_AltimeterReadPressureandTempIfActionSubsystem2I2CMasterReadWrite2
  I2C Master Read/Write3 : stm32f4_i2c_lib/I2C Master Read//Write  configuration=Transaction  module=1  lastmodule=3  transfer=Blocking  dutycycle=TLow/THigh = 2  clkspeed=400  timeout=25  writecount=1  readcount=1  sdapin=C9  sclpin=A8  waitwritetime=0  forcestop=on  inputtypearray=[2 3 3]  outputtypearray=[2 3 3]  confstr="[\"C\",\"9\",\"A\",\"8\",\"1\",\"1\",\"6\",\"0\",\"I2C_DutyCycle_2\",\"0\",\"on\"]"  sampletime=-1  sampletimestr=Inf  blockid=Baro_AltimeterReadPressureandTempIfActionSubsystem2I2CMasterReadWrite3
  If : If  IfExpression=u1 == 0  ShowElse=off
  If Action Subsystem : Subsystem  TreatAsAtomicUnit=on
  If Action Subsystem1 : Subsystem  TreatAsAtomicUnit=on
  If Action Subsystem2 : Subsystem  TreatAsAtomicUnit=on
  If1 : If  IfExpression=u1 == 0  ShowElse=off
  If2 : If  IfExpression=u1 == 0  ShowElse=off
  Shift Arithmetic1 : ArithShift  BitShiftNumber=8  BitShiftDirection=Left
  Shift Arithmetic2 : ArithShift  BitShiftNumber=6  BitShiftDirection=Right
  Shift Arithmetic9 : ArithShift  BitShiftNumber=16  BitShiftDirection=Left
  Out1 : Outport  OutDataTypeStr=uint32
  wires:
  Shift Arithmetic9/1 -> Add9/1
  Shift Arithmetic1/1 -> Add9/2
  Add9/1 -> Shift Arithmetic2/1
  Shift Arithmetic2/1 -> Out1/1
  If/1 -> If Action Subsystem/Action
  Constant1/1 -> I2C Master Read/Write3/2
  I2C Master Read/Write3/2 -> If Action Subsystem/1(In1)
  Constant2/1 -> I2C Master Read/Write1/2
  Constant/1 -> I2C Master Read/Write2/1, I2C Master Read/Write1/1, I2C Master Read/Write3/1
  Constant3/1 -> I2C Master Read/Write2/2
  I2C Master Read/Write1/2 -> If Action Subsystem1/1(In2)
  If1/1 -> If Action Subsystem1/Action
  I2C Master Read/Write2/2 -> If Action Subsystem2/1(In2)
  If2/1 -> If Action Subsystem2/Action
  If Action Subsystem/1(Out1) -> Shift Arithmetic9/1
  If Action Subsystem1/1(Out1) -> Shift Arithmetic1/1
  If Action Subsystem2/1(Out1) -> Add9/3
  I2C Master Read/Write3/1 -> If/1
  I2C Master Read/Write1/1 -> If1/1
  I2C Master Read/Write2/1 -> If2/1

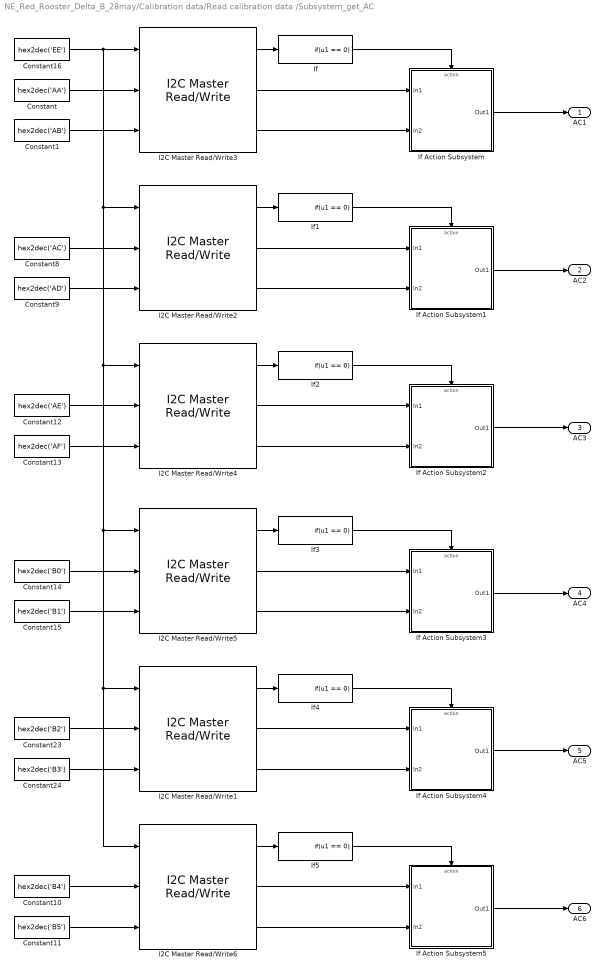
== system NE_Red_Rooster_Delta_B_28may/Calibration data/Read calibration data /Subsystem_get_AC ==
  Constant : Constant  Value=hex2dec('AA')  OutDataTypeStr=uint8
  Constant1 : Constant  Value=hex2dec('AB')  OutDataTypeStr=uint8
  Constant10 : Constant  Value=hex2dec('B4')  OutDataTypeStr=uint8
  Constant11 : Constant  Value=hex2dec('B5')  OutDataTypeStr=uint8
  Constant12 : Constant  Value=hex2dec('AE')  OutDataTypeStr=uint8
  Constant13 : Constant  Value=hex2dec('AF')  OutDataTypeStr=uint8
  Constant14 : Constant  Value=hex2dec('B0')  OutDataTypeStr=uint8
  Constant15 : Constant  Value=hex2dec('B1')  OutDataTypeStr=uint8
  Constant16 : Constant  Value=hex2dec('EE')  OutDataTypeStr=uint8
  Constant23 : Constant  Value=hex2dec('B2')  OutDataTypeStr=uint8
  Constant24 : Constant  Value=hex2dec('B3')  OutDataTypeStr=uint8
  Constant8 : Constant  Value=hex2dec('AC')  OutDataTypeStr=uint8
  Constant9 : Constant  Value=hex2dec('AD')  OutDataTypeStr=uint8
  I2C Master Read/Write1 : stm32f4_i2c_lib/I2C Master Read//Write  configuration=Transaction  module=1  lastmodule=3  transfer=Blocking  dutycycle=TLow/THigh = 2  clkspeed=400  timeout=25  writecount=2  readcount=2  sdapin=C9  sclpin=A8  waitwritetime=0  forcestop=off  inputtypearray=[3 3 3 3]  outputtypearray=[3 3 3 3]  confstr="[\"C\",\"9\",\"A\",\"8\",\"1\",\"1\",\"6\",\"0\",\"I2C_DutyCycle_2\",\"0\",\"off\"]"  sampletime=-1  sampletimestr=Inf  blockid=CalibrationdataReadcalibrationdataSubsystem_get_ACI2CMasterReadWrite1
  I2C Master Read/Write2 : stm32f4_i2c_lib/I2C Master Read//Write  configuration=Transaction  module=1  lastmodule=3  transfer=Blocking  dutycycle=TLow/THigh = 2  clkspeed=400  timeout=25  writecount=2  readcount=2  sdapin=C9  sclpin=A8  waitwritetime=0  forcestop=off  inputtypearray=[3 3 3 3]  outputtypearray=[3 3 3 3]  confstr="[\"C\",\"9\",\"A\",\"8\",\"1\",\"1\",\"6\",\"0\",\"I2C_DutyCycle_2\",\"0\",\"off\"]"  sampletime=-1  sampletimestr=Inf  blockid=CalibrationdataReadcalibrationdataSubsystem_get_ACI2CMasterReadWrite2
  I2C Master Read/Write3 : stm32f4_i2c_lib/I2C Master Read//Write  configuration=Transaction  module=1  lastmodule=3  transfer=Blocking  dutycycle=TLow/THigh = 2  clkspeed=400  timeout=25  writecount=2  readcount=2  sdapin=C9  sclpin=A8  waitwritetime=0  forcestop=off  inputtypearray=[3 3 3 3]  outputtypearray=[3 3 3 3]  confstr="[\"C\",\"9\",\"A\",\"8\",\"1\",\"1\",\"6\",\"0\",\"I2C_DutyCycle_2\",\"0\",\"off\"]"  sampletime=-1  sampletimestr=Inf  blockid=CalibrationdataReadcalibrationdataSubsystem_get_ACI2CMasterReadWrite3
  I2C Master Read/Write4 : stm32f4_i2c_lib/I2C Master Read//Write  configuration=Transaction  module=1  lastmodule=3  transfer=Blocking  dutycycle=TLow/THigh = 2  clkspeed=400  timeout=25  writecount=2  readcount=2  sdapin=C9  sclpin=A8  waitwritetime=0  forcestop=off  inputtypearray=[3 3 3 3]  outputtypearray=[3 3 3 3]  confstr="[\"C\",\"9\",\"A\",\"8\",\"1\",\"1\",\"6\",\"0\",\"I2C_DutyCycle_2\",\"0\",\"off\"]"  sampletime=-1  sampletimestr=Inf  blockid=CalibrationdataReadcalibrationdataSubsystem_get_ACI2CMasterReadWrite4
  I2C Master Read/Write5 : stm32f4_i2c_lib/I2C Master Read//Write  configuration=Transaction  module=1  lastmodule=3  transfer=Blocking  dutycycle=TLow/THigh = 2  clkspeed=400  timeout=25  writecount=2  readcount=2  sdapin=C9  sclpin=A8  waitwritetime=0  forcestop=off  inputtypearray=[3 3 3 3]  outputtypearray=[3 3 3 3]  confstr="[\"C\",\"9\",\"A\",\"8\",\"1\",\"1\",\"6\",\"0\",\"I2C_DutyCycle_2\",\"0\",\"off\"]"  sampletime=-1  sampletimestr=Inf  blockid=CalibrationdataReadcalibrationdataSubsystem_get_ACI2CMasterReadWrite5
  I2C Master Read/Write6 : stm32f4_i2c_lib/I2C Master Read//Write  configuration=Transaction  module=1  lastmodule=3  transfer=Blocking  dutycycle=TLow/THigh = 2  clkspeed=400  timeout=25  writecount=2  readcount=2  sdapin=C9  sclpin=A8  waitwritetime=0  forcestop=off  inputtypearray=[3 3 3 3]  outputtypearray=[3 3 3 3]  confstr="[\"C\",\"9\",\"A\",\"8\",\"1\",\"1\",\"6\",\"0\",\"I2C_DutyCycle_2\",\"0\",\"off\"]"  sampletime=-1  sampletimestr=Inf  blockid=CalibrationdataReadcalibrationdataSubsystem_get_ACI2CMasterReadWrite6
  If{,1..5} (6 alike) : If  IfExpression=u1 == 0  ShowElse=off
  If Action Subsystem : Subsystem  TreatAsAtomicUnit=on
  If Action Subsystem1 : Subsystem  TreatAsAtomicUnit=on
  If Action Subsystem2 : Subsystem  TreatAsAtomicUnit=on
  If Action Subsystem3 : Subsystem  TreatAsAtomicUnit=on
  If Action Subsystem4 : Subsystem  TreatAsAtomicUnit=on
  If Action Subsystem5 : Subsystem  TreatAsAtomicUnit=on
  AC1 : Outport
  AC2 : Outport  Port=2
  AC3 : Outport  Port=3
  AC4 : Outport  Port=4
  AC5 : Outport  Port=5
  AC6 : Outport  Port=6
  wires:
  I2C Master Read/Write2/1 -> If1/1
  If2/1 -> If Action Subsystem2/Action
  If Action Subsystem2/1(Out1) -> AC3/1
  I2C Master Read/Write4/2 -> If Action Subsystem2/1(In1)
  I2C Master Read/Write2/2 -> If Action Subsystem1/1(In1)
  If Action Subsystem/1(Out1) -> AC1/1
  I2C Master Read/Write3/3 -> If Action Subsystem/2(In2)
  I2C Master Read/Write4/3 -> If Action Subsystem2/2(In2)
  Constant/1 -> I2C Master Read/Write3/2
  I2C Master Read/Write3/2 -> If Action Subsystem/1(In1)
  Constant9/1 -> I2C Master Read/Write2/3
  If/1 -> If Action Subsystem/Action
  If1/1 -> If Action Subsystem1/Action
  I2C Master Read/Write4/1 -> If2/1
  Constant8/1 -> I2C Master Read/Write2/2
  Constant1/1 -> I2C Master Read/Write3/3
  Constant12/1 -> I2C Master Read/Write4/2
  Constant13/1 -> I2C Master Read/Write4/3
  I2C Master Read/Write3/1 -> If/1
  I2C Master Read/Write2/3 -> If Action Subsystem1/2(In2)
  If Action Subsystem1/1(Out1) -> AC2/1
  I2C Master Read/Write1/1 -> If4/1
  If5/1 -> If Action Subsystem5/Action
  If Action Subsystem5/1(Out1) -> AC6/1
  I2C Master Read/Write6/2 -> If Action Subsystem5/1(In1)
  I2C Master Read/Write1/2 -> If Action Subsystem4/1(In1)
  If Action Subsystem3/1(Out1) -> AC4/1
  I2C Master Read/Write5/3 -> If Action Subsystem3/2(In2)
  I2C Master Read/Write6/3 -> If Action Subsystem5/2(In2)
  Constant14/1 -> I2C Master Read/Write5/2
  I2C Master Read/Write5/2 -> If Action Subsystem3/1(In1)
  Constant24/1 -> I2C Master Read/Write1/3
  If3/1 -> If Action Subsystem3/Action
  If4/1 -> If Action Subsystem4/Action
  I2C Master Read/Write6/1 -> If5/1
  Constant23/1 -> I2C Master Read/Write1/2
  Constant15/1 -> I2C Master Read/Write5/3
  Constant10/1 -> I2C Master Read/Write6/2
  Constant11/1 -> I2C Master Read/Write6/3
  Constant16/1 -> I2C Master Read/Write3/1, I2C Master Read/Write2/1, I2C Master Read/Write5/1, I2C Master Read/Write1/1, I2C Master Read/Write6/1, I2C Master Read/Write4/1
  I2C Master Read/Write5/1 -> If3/1
  I2C Master Read/Write1/3 -> If Action Subsystem4/2(In2)
  If Action Subsystem4/1(Out1) -> AC5/1

== system NE_Red_Rooster_Delta_B_28may/Calibration data/Read calibration data /Subsystem_get_B ==
  Constant12 : Constant  Value=hex2dec('B6')  OutDataTypeStr=uint8
  Constant13 : Constant  Value=hex2dec('B7')  OutDataTypeStr=uint8
  Constant14 : Constant  Value=hex2dec('B8')  OutDataTypeStr=uint8
  Constant15 : Constant  Value=hex2dec('B9')  OutDataTypeStr=uint8
  Constant16 : Constant  Value=hex2dec('EE')  OutDataTypeStr=uint8
  I2C Master Read/Write2 : stm32f4_i2c_lib/I2C Master Read//Write  configuration=Transaction  module=1  lastmodule=3  transfer=Blocking  dutycycle=TLow/THigh = 2  clkspeed=400  timeout=25  writecount=2  readcount=2  sdapin=C9  sclpin=A8  waitwritetime=0  forcestop=off  inputtypearray=[3 3 3 3]  outputtypearray=[3 3 3 3]  confstr="[\"C\",\"9\",\"A\",\"8\",\"1\",\"1\",\"6\",\"0\",\"I2C_DutyCycle_2\",\"0\",\"off\"]"  sampletime=-1  sampletimestr=Inf  blockid=CalibrationdataReadcalibrationdataSubsystem_get_BI2CMasterReadWrite2
  I2C Master Read/Write3 : stm32f4_i2c_lib/I2C Master Read//Write  configuration=Transaction  module=1  lastmodule=3  transfer=Blocking  dutycycle=TLow/THigh = 2  clkspeed=400  timeout=25  writecount=2  readcount=2  sdapin=C9  sclpin=A8  waitwritetime=0  forcestop=off  inputtypearray=[3 3 3 3]  outputtypearray=[3 3 3 3]  confstr="[\"C\",\"9\",\"A\",\"8\",\"1\",\"1\",\"6\",\"0\",\"I2C_DutyCycle_2\",\"0\",\"off\"]"  sampletime=-1  sampletimestr=Inf  blockid=CalibrationdataReadcalibrationdataSubsystem_get_BI2CMasterReadWrite3
  If : If  IfExpression=u1 == 0  ShowElse=off
  If Action Subsystem : Subsystem  TreatAsAtomicUnit=on
  If Action Subsystem1 : Subsystem  TreatAsAtomicUnit=on
  If1 : If  IfExpression=u1 == 0  ShowElse=off
  B1 : Outport
  B2 : Outport  Port=2
  wires:
  I2C Master Read/Write2/1 -> If1/1
  I2C Master Read/Write2/2 -> If Action Subsystem1/1(In1)
  If Action Subsystem/1(Out1) -> B1/1
  I2C Master Read/Write3/3 -> If Action Subsystem/2(In2)
  I2C Master Read/Write3/2 -> If Action Subsystem/1(In1)
  If/1 -> If Action Subsystem/Action
  If1/1 -> If Action Subsystem1/Action
  Constant16/1 -> I2C Master Read/Write3/1, I2C Master Read/Write2/1
  I2C Master Read/Write3/1 -> If/1
  I2C Master Read/Write2/3 -> If Action Subsystem1/2(In2)
  If Action Subsystem1/1(Out1) -> B2/1
  Constant15/1 -> I2C Master Read/Write2/3
  Constant14/1 -> I2C Master Read/Write2/2
  Constant13/1 -> I2C Master Read/Write3/3
  Constant12/1 -> I2C Master Read/Write3/2
